simulink model "svpwm_sfunction1"  (R2022a)
settings: Solver=ode23tb  StartTime=0.0  StopTime=0.05  MaxStep=0.00001  RelTol=1e-3  EnableMultiTasking=on
libraries: simulink x1
settings Model: Creator=YUAN  LastModifiedBy=25313
settings SolverCC: AlgebraicLoopSolver=TrustRegion
settings DataIOCC: LimitDataPoints=on  SaveFormat=Array  SignalLoggingSaveFormat=ModelDataLogs  ReturnWorkspaceOutputs=off
settings OptimizationCC: ExpressionDepthLimit=2147483647  LifeSpan=inf
settings DebuggingCC: UnderspecifiedInitializationDetection=Classic  MergeDetectMultiDrivingBlocksExec=none  SolverPrmCheckMsg=warning  FcnCallInpInsideContextMsg=warning  UnconnectedInputMsg=warning  UnconnectedOutputMsg=warning  UnconnectedLineMsg=warning  StateNameClashWarn=warning  SFUnexpectedBacktrackingDiag=warning  SFNoUnconditionalDefaultTransitionDiag=warning  SFExecutionAtInitializationDiag=none  SFMachineParentedDataDiag=warning  ArithmeticOperatorsInVariantConditions=warning
settings HardwareCC: ProdBitPerPointer=32  ProdBitPerSizeT=32  ProdBitPerPtrDiffT=32  ProdLargestAtomicFloat=None  ProdIntDivRoundTo=Undefined  ProdEndianess=Unspecified  ProdWordSize=32  ProdHWDeviceType=32-bit Generic
settings ModelReferenceCC: PropagateSignalLabelsOutOfModel=off
settings SFSimCC: SimUseLocalCustomCode=off  CustomCodeUndefinedFunction=UseInterfaceOnly
settings RTWCC: RTWUseLocalCustomCode=off
settings CodeAppCC: StateflowObjectComments=on
settings GRTTargetCC: TargetLangStandard=C89/C90 (ANSI)  CombineOutputUpdateFcns=off  GRTInterface=on
settings ConfigComp: CovMetricSettings=dw  CovSaveCumulativeToWorkspaceVar=on  CovSaveSingleToWorkspaceVar=on  CovExternalEMLEnable=off

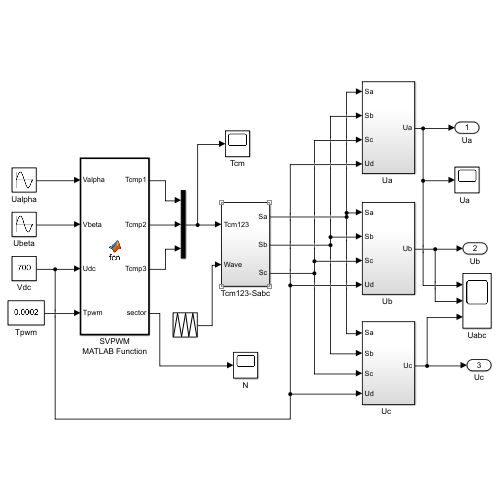
[thumbnail: Simulink's stored preview of the top-level diagram]
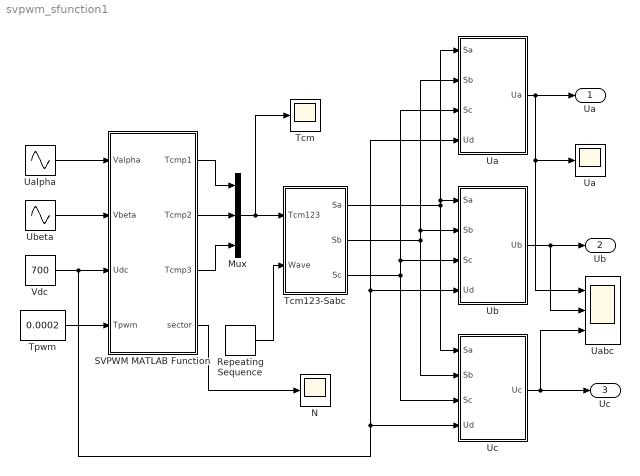
== system svpwm_sfunction1 ==
  Mux : Mux  Inputs=3
  N : Scope
  Repeating Sequence : simulink/Sources/Repeating Sequence  rep_seq_t=[0 1/10000 1/5000]  rep_seq_y=[0 1/10000 0]
  SVPWM MATLAB Function : MATLAB Function  TreatAsAtomicUnit=on
  Tcm : Scope
  Tcm123-Sabc : Subsystem
  Tpwm : Constant  Value=0.0002
  "Ua " : Subsystem
  "Ua  " : Scope
  Uabc : Scope  NumInputPorts=3
  Ualpha : Sin  Amplitude=200  Frequency=100*pi  Phase=pi/2
  "Ub " : Subsystem
  Ubeta : Sin  Amplitude=200  Frequency=100*pi
  "Uc  " : Subsystem
  Vdc : Constant  Value=700
  Ua : Outport
  Ub : Outport  Port=2
  Uc : Outport  Port=3
  wires:
  Ualpha/1 -> SVPWM MATLAB Function/1(Valpha)
  Ubeta/1 -> SVPWM MATLAB Function/2(Vbeta)
  Tpwm/1 -> SVPWM MATLAB Function/4(Tpwm)
  Mux/1 -> Tcm123-Sabc/1(Tcm123), Tcm/1
  Repeating Sequence/1 -> Tcm123-Sabc/2(Wave)
  Tcm123-Sabc/1(Sa) -> "Ua "/1(Sa), "Ub "/1(Sa), "Uc  "/1("Sa ")
  Tcm123-Sabc/2(Sb) -> "Ua "/2(Sb), "Ub "/2(Sb), "Uc  "/2(Sb)
  Tcm123-Sabc/3(Sc) -> "Ua "/3(Sc), "Ub "/3(Sc), "Uc  "/3(Sc)
  "Ua "/1(Ua) -> Uabc/1, "Ua  "/1, Ua/1
  "Ub "/1(Ub) -> Uabc/2, Ub/1
  "Uc  "/1(Uc) -> Uc/1, Uabc/3
  Vdc/1 -> "Uc  "/4(Ud), "Ua "/4(Ud), "Ub "/4(Ud), SVPWM MATLAB Function/3(Udc)
  SVPWM MATLAB Function/2(Tcmp2) -> Mux/2
  SVPWM MATLAB Function/3(Tcmp3) -> Mux/3
  SVPWM MATLAB Function/1(Tcmp1) -> Mux/1
  SVPWM MATLAB Function/4(sector) -> N/1

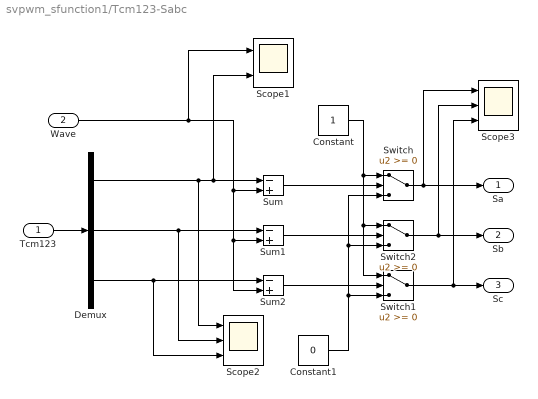
== system svpwm_sfunction1/Tcm123-Sabc ==
  Tcm123 : Inport
  Wave : Inport  Port=2
  Constant : Constant
  Constant1 : Constant  Value=0
  Demux : Demux  Outputs=3
  Scope1 : Scope  NumInputPorts=2
  Scope2 : Scope  NumInputPorts=3
  Scope3 : Scope  NumInputPorts=3
  Sum : Sum  Inputs=-+  SaturateOnIntegerOverflow=on
  Sum1 : Sum  Inputs=-+  SaturateOnIntegerOverflow=on
  Sum2 : Sum  Inputs=-+  SaturateOnIntegerOverflow=on
  Switch : Switch  InputSameDT=off
  Switch1 : Switch  InputSameDT=off
  Switch2 : Switch  InputSameDT=off
  Sa : Outport
  Sb : Outport  Port=2
  Sc : Outport  Port=3
  wires:
  Switch1/1 -> Sc/1, Scope3/3
  Switch2/1 -> Sb/1, Scope3/2
  Switch/1 -> Sa/1, Scope3/1
  Constant1/1 -> Switch1/3, Switch2/3, Switch/3
  Constant/1 -> Switch/1, Switch2/1, Switch1/1
  Sum2/1 -> Switch1/2
  Sum1/1 -> Switch2/2
  Sum/1 -> Switch/2
  Tcm123/1 -> Demux/1
  Demux/3 -> Sum2/1, Scope2/3
  Demux/2 -> Sum1/1, Scope2/2
  Demux/1 -> Scope1/2, Sum/1, Scope2/1
  Wave/1 -> Sum1/2, Sum2/2, Sum/2, Scope1/1

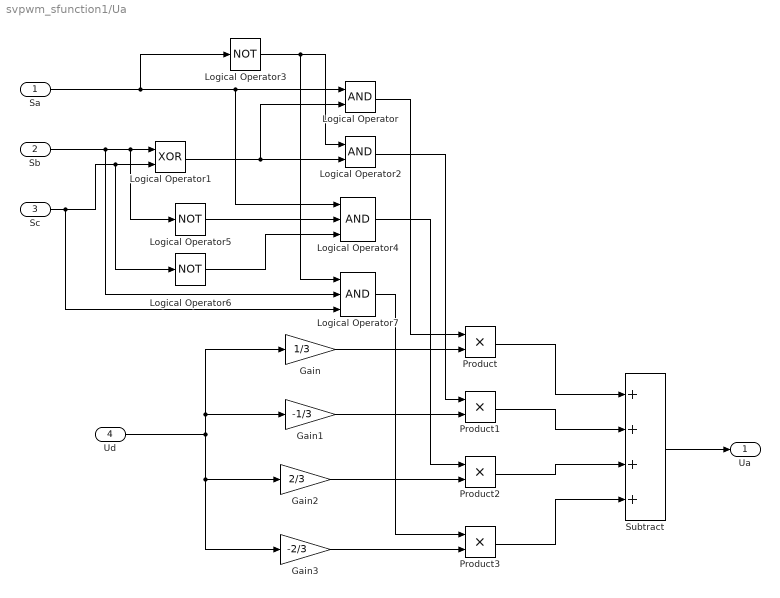
== system svpwm_sfunction1/Ua  ==
  Sa : Inport
  Sb : Inport  Port=2
  Sc : Inport  Port=3
  Ud : Inport  Port=4
  Gain : Gain  Gain=1/3
  Gain1 : Gain  Gain=-1/3
  Gain2 : Gain  Gain=2/3
  Gain3 : Gain  Gain=-2/3
  Logical Operator : Logic  AllPortsSameDT=off  OutDataTypeStr=boolean
  Logical Operator1 : Logic  Operator=XOR  AllPortsSameDT=off  OutDataTypeStr=boolean
  Logical Operator2 : Logic  AllPortsSameDT=off  OutDataTypeStr=boolean
  Logical Operator3 : Logic  Operator=NOT  AllPortsSameDT=off  OutDataTypeStr=boolean
  Logical Operator4 : Logic  Inputs=3  AllPortsSameDT=off  OutDataTypeStr=boolean
  Logical Operator5 : Logic  Operator=NOT  AllPortsSameDT=off  OutDataTypeStr=boolean
  Logical Operator6 : Logic  Operator=NOT  AllPortsSameDT=off  OutDataTypeStr=boolean
  Logical Operator7 : Logic  Inputs=3  AllPortsSameDT=off  OutDataTypeStr=boolean
  Product{,1..3} (4 alike) : Product  RndMeth=Zero
  Subtract : Sum  Inputs=++++
  Ua : Outport
  wires:
  Ud/1 -> Gain3/1, Gain2/1, Gain1/1, Gain/1
  Gain/1 -> Product/2
  Gain1/1 -> Product1/2
  Gain2/1 -> Product2/2
  Gain3/1 -> Product3/2
  Product/1 -> Subtract/1
  Product1/1 -> Subtract/2
  Product2/1 -> Subtract/3
  Product3/1 -> Subtract/4
  Subtract/1 -> Ua/1
  Logical Operator/1 -> Product/1
  Sa/1 -> Logical Operator4/1, Logical Operator/1, Logical Operator3/1
  Sb/1 -> Logical Operator7/2, Logical Operator5/1, Logical Operator1/1
  Sc/1 -> Logical Operator7/3, Logical Operator6/1, Logical Operator1/2
  Logical Operator1/1 -> Logical Operator/2, Logical Operator2/2
  Logical Operator2/1 -> Product1/1
  Logical Operator3/1 -> Logical Operator2/1, Logical Operator7/1
  Logical Operator4/1 -> Product2/1
  Logical Operator5/1 -> Logical Operator4/2
  Logical Operator6/1 -> Logical Operator4/3
  Logical Operator7/1 -> Product3/1

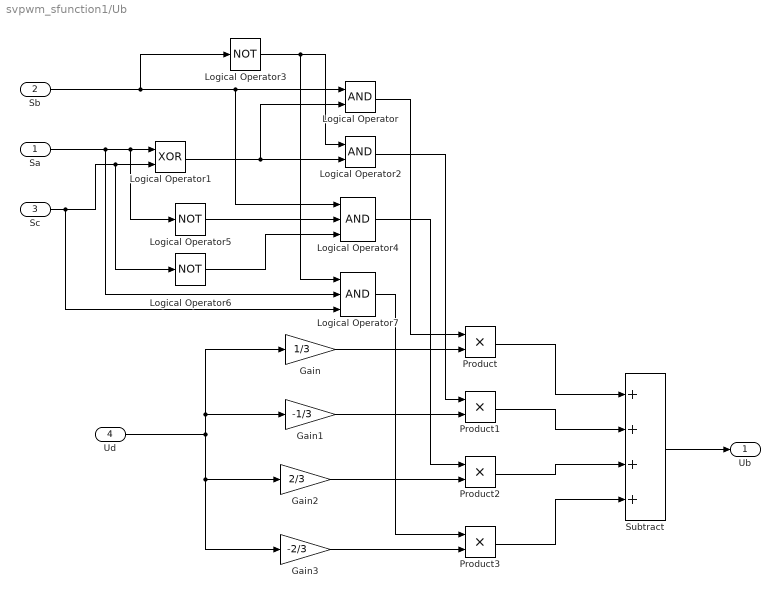
== system svpwm_sfunction1/Ub  ==
  Sa : Inport
  Sb : Inport  Port=2
  Sc : Inport  Port=3
  Ud : Inport  Port=4
  Gain : Gain  Gain=1/3
  Gain1 : Gain  Gain=-1/3
  Gain2 : Gain  Gain=2/3
  Gain3 : Gain  Gain=-2/3
  Logical Operator : Logic  AllPortsSameDT=off  OutDataTypeStr=boolean
  Logical Operator1 : Logic  Operator=XOR  AllPortsSameDT=off  OutDataTypeStr=boolean
  Logical Operator2 : Logic  AllPortsSameDT=off  OutDataTypeStr=boolean
  Logical Operator3 : Logic  Operator=NOT  AllPortsSameDT=off  OutDataTypeStr=boolean
  Logical Operator4 : Logic  Inputs=3  AllPortsSameDT=off  OutDataTypeStr=boolean
  Logical Operator5 : Logic  Operator=NOT  AllPortsSameDT=off  OutDataTypeStr=boolean
  Logical Operator6 : Logic  Operator=NOT  AllPortsSameDT=off  OutDataTypeStr=boolean
  Logical Operator7 : Logic  Inputs=3  AllPortsSameDT=off  OutDataTypeStr=boolean
  Product{,1..3} (4 alike) : Product  RndMeth=Zero
  Subtract : Sum  Inputs=++++
  Ub : Outport
  wires:
  Ud/1 -> Gain3/1, Gain2/1, Gain1/1, Gain/1
  Gain/1 -> Product/2
  Gain1/1 -> Product1/2
  Gain2/1 -> Product2/2
  Gain3/1 -> Product3/2
  Product/1 -> Subtract/1
  Product1/1 -> Subtract/2
  Product2/1 -> Subtract/3
  Product3/1 -> Subtract/4
  Subtract/1 -> Ub/1
  Logical Operator/1 -> Product/1
  Sb/1 -> Logical Operator4/1, Logical Operator/1, Logical Operator3/1
  Sa/1 -> Logical Operator7/2, Logical Operator5/1, Logical Operator1/1
  Sc/1 -> Logical Operator7/3, Logical Operator6/1, Logical Operator1/2
  Logical Operator1/1 -> Logical Operator/2, Logical Operator2/2
  Logical Operator2/1 -> Product1/1
  Logical Operator3/1 -> Logical Operator2/1, Logical Operator7/1
  Logical Operator4/1 -> Product2/1
  Logical Operator5/1 -> Logical Operator4/2
  Logical Operator6/1 -> Logical Operator4/3
  Logical Operator7/1 -> Product3/1

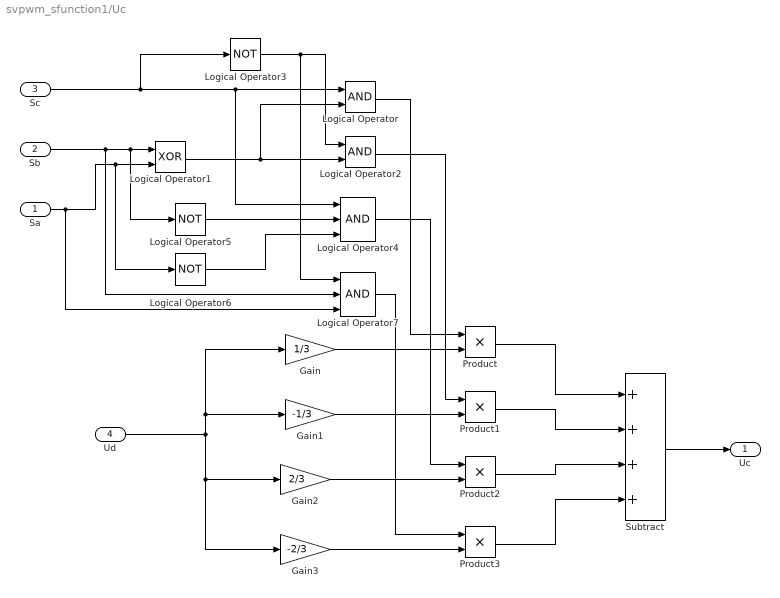
== system svpwm_sfunction1/Uc   ==
  "Sa " : Inport
  Sb : Inport  Port=2
  Sc : Inport  Port=3
  Ud : Inport  Port=4
  Gain : Gain  Gain=1/3
  Gain1 : Gain  Gain=-1/3
  Gain2 : Gain  Gain=2/3
  Gain3 : Gain  Gain=-2/3
  Logical Operator : Logic  AllPortsSameDT=off  OutDataTypeStr=boolean
  Logical Operator1 : Logic  Operator=XOR  AllPortsSameDT=off  OutDataTypeStr=boolean
  Logical Operator2 : Logic  AllPortsSameDT=off  OutDataTypeStr=boolean
  Logical Operator3 : Logic  Operator=NOT  AllPortsSameDT=off  OutDataTypeStr=boolean
  Logical Operator4 : Logic  Inputs=3  AllPortsSameDT=off  OutDataTypeStr=boolean
  Logical Operator5 : Logic  Operator=NOT  AllPortsSameDT=off  OutDataTypeStr=boolean
  Logical Operator6 : Logic  Operator=NOT  AllPortsSameDT=off  OutDataTypeStr=boolean
  Logical Operator7 : Logic  Inputs=3  AllPortsSameDT=off  OutDataTypeStr=boolean
  Product{,1..3} (4 alike) : Product  RndMeth=Zero
  Subtract : Sum  Inputs=++++
  Uc : Outport
  wires:
  Ud/1 -> Gain3/1, Gain2/1, Gain1/1, Gain/1
  Gain/1 -> Product/2
  Gain1/1 -> Product1/2
  Gain2/1 -> Product2/2
  Gain3/1 -> Product3/2
  Product/1 -> Subtract/1
  Product1/1 -> Subtract/2
  Product2/1 -> Subtract/3
  Product3/1 -> Subtract/4
  Subtract/1 -> Uc/1
  Logical Operator/1 -> Product/1
  Sc/1 -> Logical Operator4/1, Logical Operator/1, Logical Operator3/1
  Sb/1 -> Logical Operator7/2, Logical Operator5/1, Logical Operator1/1
  "Sa "/1 -> Logical Operator7/3, Logical Operator6/1, Logical Operator1/2
  Logical Operator1/1 -> Logical Operator/2, Logical Operator2/2
  Logical Operator2/1 -> Product1/1
  Logical Operator3/1 -> Logical Operator2/1, Logical Operator7/1
  Logical Operator4/1 -> Product2/1
  Logical Operator5/1 -> Logical Operator4/2
  Logical Operator6/1 -> Logical Operator4/3
  Logical Operator7/1 -> Product3/1

== matlab function svpwm_sfunction1/SVPWM MATLAB Function ==
  data: Valpha input; Tcmp1 output; Vbeta input; Tcmp2 output; Tcmp3 output; Udc input; Tpwm input; sector output
function [Tcmp1,Tcmp2,Tcmp3,sector] = fcn(Valpha,Vbeta,Udc,Tpwm)
%#codegen

sector = 0;
Tcmp1 = 0;
Tcmp2 = 0;
Tcmp3 = 0;

%========Parameters statement================

    Vref1 = Vbeta;							                   
    Vref2 = (sqrt(3)*Valpha - Vbeta)/2; 				    
    Vref3 = (-sqrt(3)*Valpha - Vbeta)/2;					
   
 %========Sector calculation=================

  if (Vref1>0)
	   sector = 1;
  end
  if (Vref2>0)
	   sector = sector+2;
  end
  if (Vref3>0)
       sector = sector+4;
  end

%======== X Y Z calculation===================

X = sqrt(3)*Vbeta*Tpwm/Udc;
Y = Tpwm/Udc*(3/2*Valpha+sqrt(3)/2*Vbeta);
Z = Tpwm/Udc*(-3/2*Valpha+sqrt(3)/2*Vbeta);	         

%==========Duty ratio calculation================
switch (sector)   
    case 1
        T1 = Z; T2 = Y; 
	case 2
        T1 = Y; T2 = -X; 
	case 3
        T1 = -Z; T2 = X; 
	case 4
        T1 = -X; T2 = Z;
	case 5
        T1 = X; T2 = -Y;
    otherwise
        T1 = -Y; T2 = -Z;
end

if T1+T2 > Tpwm
    T1 = T1/(T1+T2);
    T2 = T2/(T1+T2);
else
    T1 = T1;
    T2 = T2;
end
ta = (Tpwm-(T1+T2))/4.0;
tb = ta+T1/2;
tc = tb+T2/2;

%==========Duty ratio calculation================
switch (sector)
    case 1 
        Tcmp1=tb;
        Tcmp2=ta;
        Tcmp3=tc; 
        
    case 2 
        Tcmp1=ta;
        Tcmp2=tc;
        Tcmp3=tb; 
       
    case 3 
        Tcmp1=ta;
        Tcmp2=tb;
        Tcmp3=tc; 
        
    case 4 
        Tcmp1=tc;
        Tcmp2=tb;
        Tcmp3=ta;
        
    case 5 
        Tcmp1=tc;
        Tcmp2=ta;
        Tcmp3=tb;
        
   case 6
       Tcmp1=tb;
       Tcmp2=tc;
       Tcmp3=ta;
end
end
